simulink model "AAI"  (R2021a)
settings: Solver=FixedStepAuto  StartTime=0.0  StopTime=10.0  FixedStep=1e-4  RelTol=1e-3  EnableMultiTasking=on
undefined symbols (not defined in the file): D0, D1, PTC16, PTC17
libraries: frdmk64flib x3
settings Model: ExtModeTrigDuration=5  Creator=majet  LastModifiedBy=majet
settings OptimizationCC: EnhancedBackFolding=on  PassReuseOutputArgsAs=Individual arguments  ZeroExternalMemoryAtStartup=off  ZeroInternalMemoryAtStartup=off  MaxStackSize=64  OptimizeBlockOrder=speed  DifferentSizesBufferReuse=on  OptimizationCustomize=off  EfficientTunableParamExpr=on
settings DebuggingCC: ParameterTunabilityLossMsg=error
settings HardwareCC: ProdBitPerPointer=32  ProdBitPerSizeT=32  ProdBitPerPtrDiffT=32  ProdLargestAtomicInteger=Long  ProdLargestAtomicFloat=Double  ProdWordSize=32  ProdHWDeviceType=ARM Compatible->ARM Cortex
settings SFSimCC: MATLABDynamicMemAlloc=off
settings RTWCC: SystemTargetFile=ert.tlc  HardwareBoard=NXP FRDM-K64F  TLCOptions="-aInlineSetEventsForThisBaseRateFcn=TLC_FALSE -aSuppressMultiTaskScheduler=TLC_FALSE  -aRateBasedStepFcn=0"  TemplateMakefile=ert_default_tmf  Toolchain=GNU Tools for ARM Embedded Processors
settings CodeAppCC: ForceParamTrailComments=on  IgnoreCustomStorageClasses=off  OperatorAnnotations=on  SimulinkDataObjDesc=on  SFDataObjDesc=on  InsertBlockDesc=on
settings ERTTargetCC: ExtModeTransport=4  ExtModeMexFile=sendToCommService

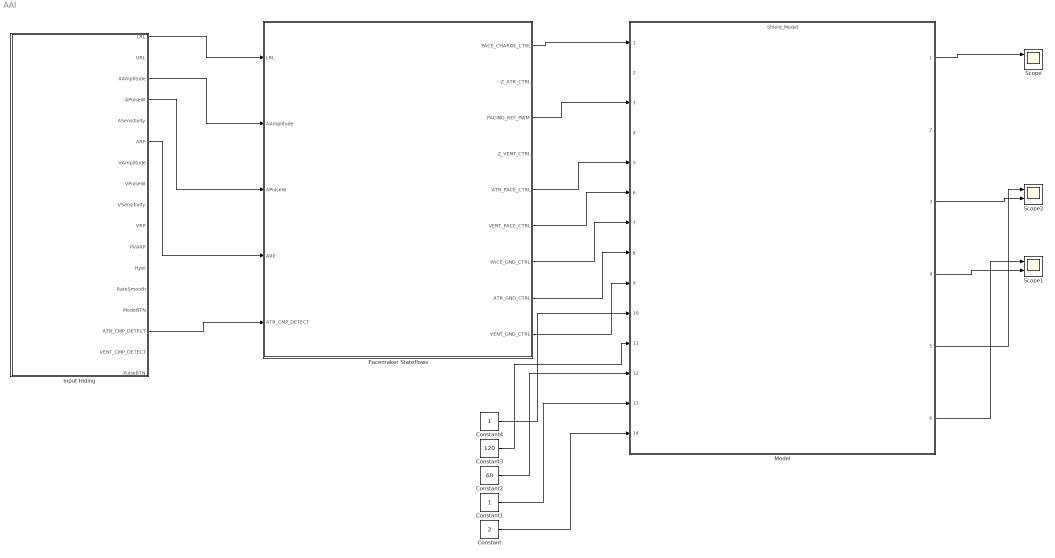
== system AAI ==
  Constant : Constant  Value=2
  Constant1 : Constant
  Constant2 : Constant  Value=60
  Constant3 : Constant  Value=120
  Constant4 : Constant  OutDataTypeStr=boolean
  Input Hiding : Subsystem
  Model : ModelReference  ModelNameDialog=Shield_Model.slxp  ModelReferenceVersion=1.25  CopyOfModelProtected=on
  Pacemaker Stateflows : Stateflow chart  TreatAsAtomicUnit=on
  Scope : Scope  NumInputPorts=2
  Scope1 : Scope  NumInputPorts=2
  Scope2 : Scope  NumInputPorts=2
  wires:
  Input Hiding/4(APulseW) -> Pacemaker Stateflows/3(APulseW)
  Input Hiding/15(ATR_CMP_DETECT) -> Pacemaker Stateflows/5(ATR_CMP_DETECT)
  Input Hiding/3(AAmplitude) -> Pacemaker Stateflows/2(AAmplitude)
  Input Hiding/1(LRL) -> Pacemaker Stateflows/1(LRL)
  Input Hiding/6(ARP) -> Pacemaker Stateflows/4(ARP)
  Model/3 -> Scope2/2
  Model/6 -> Scope1/1
  Model/1 -> Scope/1
  Model/4 -> Scope1/2
  Model/5 -> Scope2/1
  Pacemaker Stateflows/1(PACE_CHARGE_CTRL) -> Model/1
  Pacemaker Stateflows/9(VENT_GND_CTRL) -> Model/9
  Pacemaker Stateflows/8(ATR_GND_CTRL) -> Model/8
  Pacemaker Stateflows/7(PACE_GND_CTRL) -> Model/7
  Pacemaker Stateflows/6(VENT_PACE_CTRL) -> Model/6
  Pacemaker Stateflows/5(ATR_PACE_CTRL) -> Model/5
  Pacemaker Stateflows/3(PACING_REF_PWM) -> Model/3
  Constant4/1 -> Model/10
  Constant3/1 -> Model/11
  Constant2/1 -> Model/12
  Constant1/1 -> Model/13
  Constant/1 -> Model/14

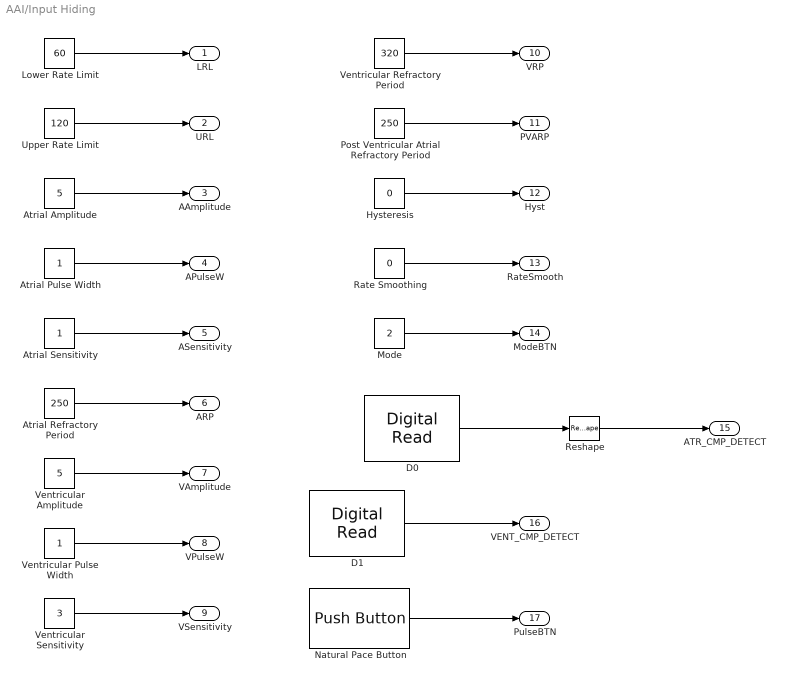
== system AAI/Input Hiding ==
  Atrial Amplitude : Constant  Value=5  OutDataTypeStr=double
  Atrial Pulse Width : Constant  OutDataTypeStr=double
  Atrial Refractory Period : Constant  Value=250  OutDataTypeStr=double
  Atrial Sensitivity : Constant  OutDataTypeStr=double
  D0 : frdmk64flib/Digital Read  Whichpin=PTC16 (D0)  SampleTime=-1
  D1 : frdmk64flib/Digital Read  Whichpin=PTC17 (D1)  SampleTime=-1
  Hysteresis : Constant  Value=0  OutDataTypeStr=double
  Lower Rate Limit : Constant  Value=60  OutDataTypeStr=double
  Mode : Constant  Value=2  OutDataTypeStr=double
  Natural Pace Button : frdmk64flib/Push Button  Whichswitch=SW3  SampleTime1=-1
  Post Ventricular Atrial Refractory Period : Constant  Value=250  OutDataTypeStr=double
  Rate Smoothing : Constant  Value=0  OutDataTypeStr=double
  Reshape : Reshape  OutputDimensionality=Customize  OutputDimensions=1
  Upper Rate Limit : Constant  Value=120  OutDataTypeStr=double
  Ventricular Amplitude : Constant  Value=5  OutDataTypeStr=double
  Ventricular Pulse Width : Constant  OutDataTypeStr=double
  Ventricular Refractory Period : Constant  Value=320  OutDataTypeStr=double
  Ventricular Sensitivity : Constant  Value=3  OutDataTypeStr=double
  LRL : Outport  OutDataTypeStr=double
  URL : Outport  Port=2  OutDataTypeStr=double
  AAmplitude : Outport  Port=3  OutDataTypeStr=double
  APulseW : Outport  Port=4  OutDataTypeStr=double
  ASensitivity : Outport  Port=5  OutDataTypeStr=double
  ARP : Outport  Port=6  OutDataTypeStr=double
  VAmplitude : Outport  Port=7  OutDataTypeStr=double
  VPulseW : Outport  Port=8  OutDataTypeStr=double
  VSensitivity : Outport  Port=9  OutDataTypeStr=double
  VRP : Outport  Port=10  OutDataTypeStr=double
  PVARP : Outport  Port=11  OutDataTypeStr=double
  Hyst : Outport  Port=12  OutDataTypeStr=double
  RateSmooth : Outport  Port=13  OutDataTypeStr=double
  ModeBTN : Outport  Port=14  OutDataTypeStr=double
  ATR_CMP_DETECT : Outport  Port=15  OutDataTypeStr=boolean
  VENT_CMP_DETECT : Outport  Port=16  OutDataTypeStr=boolean
  PulseBTN : Outport  Port=17  OutDataTypeStr=boolean
  wires:
  Lower Rate Limit/1 -> LRL/1
  Upper Rate Limit/1 -> URL/1
  Atrial Amplitude/1 -> AAmplitude/1
  Ventricular Amplitude/1 -> VAmplitude/1
  Atrial Pulse Width/1 -> APulseW/1
  Ventricular Pulse Width/1 -> VPulseW/1
  Atrial Sensitivity/1 -> ASensitivity/1
  Ventricular Sensitivity/1 -> VSensitivity/1
  Ventricular Refractory Period/1 -> VRP/1
  Atrial Refractory Period/1 -> ARP/1
  D1/1 -> VENT_CMP_DETECT/1
  Post Ventricular Atrial Refractory Period/1 -> PVARP/1
  Hysteresis/1 -> Hyst/1
  Rate Smoothing/1 -> RateSmooth/1
  Natural Pace Button/1 -> PulseBTN/1
  Mode/1 -> ModeBTN/1
  D0/1 -> Reshape/1
  Reshape/1 -> ATR_CMP_DETECT/1

== stateflow chart AAI/Pacemaker Stateflows ==
  state ENTRY
    entry:
    VENT_PACE_CTRL = 0; VENT_GND_CTRL = 0; PACE_GND_CTRL = 1;
    Z_VENT_CTRL = 0; Z_ATR_CTRL = 0; PACING_REF_PWM = AAmplitude*20;
  state PACE_ATR
    %Discharge
    entry:
    PACE_CHARGE_CTRL = 0;
    ATR_GND_CTRL = 0;
    ATR_PACE_CTRL = 1;
  state C22_CHARGE
    entry:
    ATR_PACE_CTRL = 0;
    ATR_GND_CTRL = 1;
    PACE_CHARGE_CTRL = 1;
  state INTERMEDIATE
    %In between state
    entry:
    PACE_CHARGE_CTRL = 1;
    ATR_GND_CTRL = 1;
    ATR_PACE_CTRL = 0;
  (default) -> ENTRY
  ENTRY -> C22_CHARGE
  C22_CHARGE -> PACE_ATR [order 1] : after((60000/LRL)-APulseW-ARP,msec)
  C22_CHARGE -> INTERMEDIATE [order 2] : [ATR_CMP_DETECT == high]{after(LRL,msec)}
  INTERMEDIATE -> C22_CHARGE : after(ARP,msec)
  PACE_ATR -> INTERMEDIATE : after(APulseW,msec)
  data: LRL input double; AAmplitude input double; APulseW input double; PACE_CHARGE_CTRL output double; Z_ATR_CTRL output double; PACING_REF_PWM output double; Z_VENT_CTRL output double; ATR_PACE_CTRL output double; VENT_PACE_CTRL output double; PACE_GND_CTRL output double; ATR_GND_CTRL output double; VENT_GND_CTRL output double; ARP input double; ATR_CMP_DETECT input boolean; high local boolean =true
